simulink model "Maglev_NMPC_offsetFree"  (R2025a)
settings: Solver=ode23t  StartTime=0.0  StopTime=T_sim  FixedStep=mpc.Ts  MaxStep=0.0001  RelTol=1e-4
PreLoadFcn:
  | modelPath = fileparts(which(bdroot));
  | projectRoot = fileparts(modelPath);
  | 
  | run(fullfile(projectRoot, 'setup_sim_params.m'));
  | load(fullfile(projectRoot, 'Controller_Params', 'LKFData.mat'));
  | load(fullfile(projectRoot, 'Controller_Params', 'OffsetFreeNMPCData.mat'));
  | % Add the generated code folder so Simulink can find the mexw64
  | addpath(fullfile(projectRoot, 'Controller_Design/design_nmpc_offsetfree/c_generated_code'))
  | addpath(fullfile(projectRoot, 'Controller_Design/design_nmpc_offsetfree/c_generated_code/MaglevAug_model'))
  | 
  | load('sfun_port_names')
undefined symbols (not defined in the file): airgap_soll, Ext_Fina_Val, Ext_Init_Val, grav, I_max, I_min, lkf_params, mass, nmpc, T_stp
libraries: fl_lib x11, nesl_utility x4
settings Model: Creator=Polarstern  LastModifiedBy=CelestialAurora

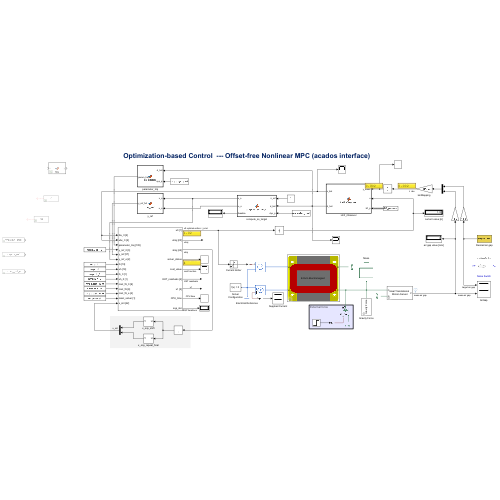
[thumbnail: Simulink's stored preview of the top-level diagram]
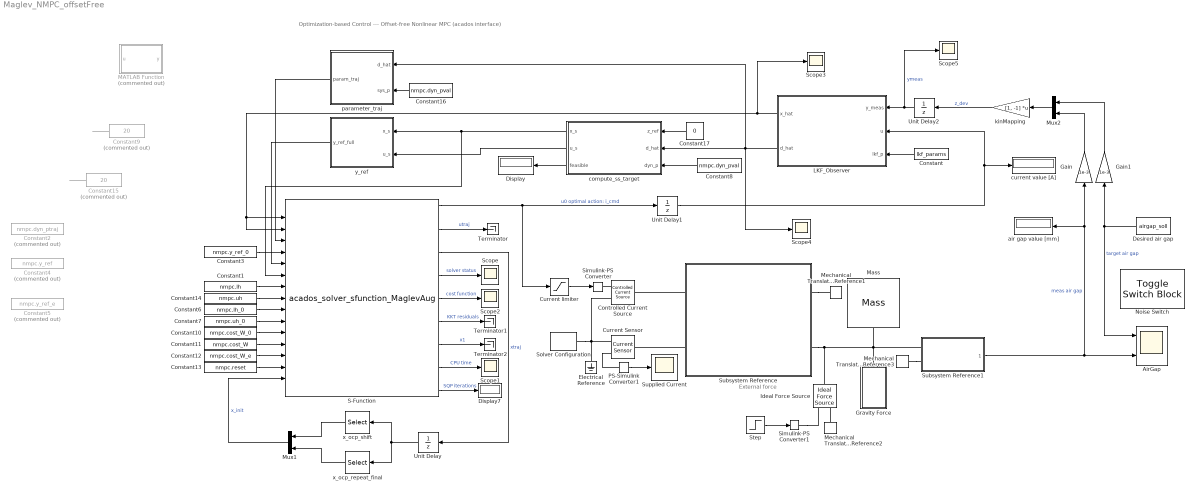
== system Maglev_NMPC_offsetFree ==
  note: Optimization-based Control --- Offset-free Nonlinear MPC (acados interface)
  note: External force
  AirGap : Scope  NumInputPorts=2
      settings: ActiveDisplayYMinimum=-0.31249999999999994  ActiveDisplayYMaximum=2.8125
  Constant : Constant  Value=lkf_params  OutDataTypeStr=Bus: lkf_Bus
  Constant1 : Constant  Value=nmpc.lh
  Constant10 : Constant  Value=nmpc.cost_W_0
  Constant11 : Constant  Value=nmpc.cost_W
  Constant12 : Constant  Value=nmpc.cost_W_e
  Constant13 : Constant  Value=nmpc.reset
  Constant14 : Constant  Value=nmpc.uh
  Constant15 : Constant  Commented=on  Value=20
  Constant16 : Constant  Value=nmpc.dyn_pval
  Constant17 : Constant  Value=0
  Constant2 : Constant  Commented=on  Value=nmpc.dyn_ptraj
  Constant3 : Constant  Value=nmpc.y_ref_0
  Constant4 : Constant  Commented=on  Value=nmpc.y_ref
  Constant5 : Constant  Commented=on  Value=nmpc.y_ref_e
  Constant6 : Constant  Value=nmpc.lh_0
  Constant7 : Constant  Value=nmpc.uh_0
  Constant8 : Constant  Value=nmpc.dyn_pval
  Constant9 : Constant  Commented=on  Value=20
  Controlled Current Source : fl_lib/Electrical/Electrical Sources/Controlled Current Source
  Current Sensor : fl_lib/Electrical/Electrical Sensors/Current Sensor
  Current limiter : Saturate  UpperLimit=I_max  LowerLimit=I_min
  Desired air gap : Constant  Value=airgap_soll
  Display : Display
  Display7 : Display
  Electrical Reference : fl_lib/Electrical/Electrical Elements/Electrical Reference
  Gain : Gain  Gain=1e-3
  Gain1 : Gain  Gain=1e-3
  Gravity Force : Subsystem
      mask DialogControl DescGroupVar Prompt: Gravity Force
      mask DialogControl DescTextVar Prompt: Fg = Mass*grav, as constant parameters predefined
      mask DialogControl DescTextVar2 Prompt: Direction: Downward
      mask Display: disp("Gravity Force")
  Ideal Force Source : fl_lib/Mechanical/Mechanical Sources/Ideal Force Source
  LKF_Observer : MATLAB Function  TreatAsAtomicUnit=on
  MATLAB Function : MATLAB Function  Commented=on  TreatAsAtomicUnit=on
  Mass : fl_lib/Mechanical/Translational Elements/Mass  mass=mass kg  num_ports=foundation.enum.numPorts2.one  v_specify=on  v_priority=Low  v=0 m/s  v_nominal_specify=off  v_nominal_value=1  v_nominal_unit=m/s  f_specify=off  f_priority=None  f=0 N  f_nominal_specify=off  f_nominal_value=700  f_nominal_unit=N
  Mechanical Translational Reference1 : fl_lib/Mechanical/Translational Elements/Mechanical Translational Reference
  Mechanical Translational Reference2 : fl_lib/Mechanical/Translational Elements/Mechanical Translational Reference
  Mechanical Translational Reference3 : fl_lib/Mechanical/Translational Elements/Mechanical Translational Reference
  Mux1 : Mux  Inputs=2
  Mux2 : Mux  Inputs=2
  Noise Switch : ToggleSwitchBlock
  PS-Simulink Converter1 : nesl_utility/PS-Simulink Converter  PhysicalDomain=network_engine_domain  SubClassName=ps_output  LeftPortType=input  RightPortType=output  PseudoPeriodic=off  Frequencies=[]  VectorFormat=inherit  Unit=inherit  AffineConversion=off
  S-Function : S-Function  FunctionName=acados_solver_sfunction_MaglevAug  SFunctionDeploymentMode=off  EnableBusSupport=off
      mask Display:
      | global sfun_input_names sfun_output_names
      | for i = 1:length(sfun_input_names)
      | 	port_label('input', i, sfun_input_names{i})
      | end
      | for i = 1:length(sfun_output_names)
      | 	port_label('output', i, sfun_output_names{i})
      | end
  Scope{,1..5} (6 alike) : Scope
      Scope settings: ActiveDisplayYMinimum=-0.49999999999999989  ActiveDisplayYMaximum=4.5
      Scope1 settings: ActiveDisplayYMinimum=-0.002376549999999999  ActiveDisplayYMaximum=0.029782950000000002  DataLoggingVariableName=ScopeData2
      Scope2 settings: ActiveDisplayYMinimum=-1  ActiveDisplayYMaximum=1  DataLoggingVariableName=ScopeData4
      Scope3 settings: ActiveDisplayYMinimum=-0.12370605676276082  ActiveDisplayYMaximum=0.39152289519586231  DataLoggingVariableName=ScopeData5
      Scope4 settings: ActiveDisplayYMinimum=-1.3296662204714107  ActiveDisplayYMaximum=0.14858706613408232  DataLoggingVariableName=ScopeData6
      Scope5 settings: ActiveDisplayYMinimum=-0.00081250000000000007  ActiveDisplayYMaximum=0.0023125000000000003  DataLoggingVariableName=ScopeData7
  Simulink-PS Converter : nesl_utility/Simulink-PS Converter  PhysicalDomain=network_engine_domain  SubClassName=ps_input  LeftPortType=input  RightPortType=output  PseudoPeriodic=off  Frequencies=[]  NoiseDistribution=none  NoiseParameters=[]  Unit=1  AffineConversion=off  FilteringAndDerivatives=zero  SimscapeFilterOrder=1  InputFilterTimeConstant=0.001  UdotUserProvided=0
  Simulink-PS Converter1 : nesl_utility/Simulink-PS Converter  PhysicalDomain=network_engine_domain  SubClassName=ps_input  LeftPortType=input  RightPortType=output  PseudoPeriodic=off  Frequencies=[]  NoiseDistribution=none  NoiseParameters=[]  Unit=1  AffineConversion=off  FilteringAndDerivatives=provide  SimscapeFilterOrder=1  InputFilterTimeConstant=0.001  UdotUserProvided=0
  Solver Configuration : nesl_utility/Solver Configuration  PhysicalDomain=network_engine_domain  SubClassName=solver  LeftPortType=input  RightPortType=generic  Tones=[]  Harmonics=[]  SimulateNoise=off  Profile=off  UseLocalSampling=off  EnableSwitchedLinearOptims=on  FrequencyDomain=off  UseCCode=off  RelTol=0.001  AbsTol=1e-06  MinStep=1e-09  ToWorkspace=off  RevertToSquareIcSolve=off  NumHomotopyIterations=100  PhasorMode=off  PhasorModeNumHarmonics=1  ConsistencySolver=NEWTON_XTOL_AFTER_FTOL  IndexReductionMethod=DerivativeReplacement  DoDC=off  ResidualTolerance=1e-09  ConsistencyTolSource=GLOBAL  ConsistencyAbsTol=0.001  ConsistencyRelTol=0.001  ConsistencyTolFactor=0.001  UseLocalSolver=off  LocalSolverChoice=NE_BACKWARD_EULER_ADVANCER  ResolveIndetEquations=on  FunctionEvalNumThread=1  LocalSolverSampleTime=0.001  DoFixedCost=off  MaxNonlinIter=3  MaxModeIter=2  ComputeImpulses=off  ImpulseIterations=2  LinearAlgebra=auto  LinearAlgebraNumThread=0  EquationFormulation=NE_TIME_EF  DelaysMemoryBudget=1024  AutomaticFiltering=on  FilteringTimeConstant=0.001  PartitionStorageMethod=AS_NEEDED  PartitionMemoryBudget=1024  PartitionMethod=ROBUST  MultibodyUseLocalSolver=off  MultibodyLocalSolverChoice=ODE1  MultibodyLocalSolverSampleTime=0.001
  Step : Step  Time=T_stp  Before=Ext_Init_Val  After=Ext_Fina_Val  SampleTime=0
  Subsystem Reference : Subsystem  ReferencedSubsystem=IntegratedElectromagnet  l_airgap=airgap_init
  Subsystem Reference1 : Subsystem  ReferencedSubsystem=IdealTrans_MotionSensor  ns_sw=isNoiseActive  ns_pw=NoisePower  ts=Ts  init_pos=airgap_init
  Supplied Current : Scope
      settings: ActiveDisplayYMinimum=-0.5608888953934309  ActiveDisplayYMaximum=6.1901533618851614  DataLoggingVariableName=ScopeData3
  Terminator : Terminator
  Terminator1 : Terminator
  Terminator2 : Terminator
  Unit Delay : UnitDelay  InitialCondition=nmpc.x_init  SampleTime=-1  HasFrameUpgradeWarning=on
  Unit Delay1 : UnitDelay  InitialCondition=lkf_params.u_eq  SampleTime=-1  HasFrameUpgradeWarning=on
  Unit Delay2 : UnitDelay  InitialCondition=nmpc.x_init_con(1)  SampleTime=-1  HasFrameUpgradeWarning=on
  air gap value [mm] : Display
      settings: Decimation=4
  compute_ss_target : MATLAB Function  TreatAsAtomicUnit=on
  current value [A] : Display
  kinMapping : Gain  Gain=[1, -1]  Multiplication=Matrix(K*u) (u vector)
  parameter_traj : MATLAB Function  TreatAsAtomicUnit=on
  x_ocp_repeat_final : Selector  IndexMode=Zero-based  InputPortWidth=(nmpc.N+1)*nmpc.nx  IndexOptions=Starting index (dialog)  Indices=nmpc.N*nmpc.nx  OutputSizes=nmpc.nx
  x_ocp_shift : Selector  IndexMode=Zero-based  InputPortWidth=(nmpc.N+1)*nmpc.nx  IndexOptions=Starting index (dialog)  Indices=nmpc.nx  OutputSizes=nmpc.N*nmpc.nx
  y_ref : MATLAB Function  TreatAsAtomicUnit=on
  wires:
  Current limiter/1 -> Simulink-PS Converter/1
  PS-Simulink Converter1/1 -> Supplied Current/1
  S-Function/1 -> Current limiter/1, Unit Delay1/1  "u0 optimal action: i_cmd"
  S-Function/2 -> Terminator/1  "utraj"
  S-Function/3 -> Unit Delay/1  "xtraj"
  S-Function/4 -> Scope/1  "solver status"
  S-Function/5 -> Scope2/1  "cost function"
  S-Function/6 -> Terminator1/1  "KKT residuals"
  S-Function/7 -> Terminator2/1  "x1"
  S-Function/8 -> Scope1/1  "CPU time"
  S-Function/9 -> Display7/1  "SQP iterations"
  Unit Delay/1 -> x_ocp_repeat_final/1, x_ocp_shift/1
  x_ocp_repeat_final/1 -> Mux1/2
  x_ocp_shift/1 -> Mux1/1
  Step/1 -> Simulink-PS Converter1/1
  LKF_Observer/1(x_hat) -> Scope3/1, S-Function/1, S-Function/2
  Constant3/1 -> S-Function/4
  Constant1/1 -> S-Function/7
  Constant14/1 -> S-Function/8
  Constant6/1 -> S-Function/9
  Constant7/1 -> S-Function/10
  Constant10/1 -> S-Function/11
  Constant11/1 -> S-Function/12
  Constant12/1 -> S-Function/13
  Constant13/1 -> S-Function/14
  Mux1/1 -> S-Function/15  "x_init"
  Gain/1 -> Mux2/2
  Subsystem Reference1/1 -> AirGap/2, air gap value [mm]/1, Gain/1  "meas air gap"
  Desired air gap/1 -> AirGap/1, Gain1/1  "target air gap"
  kinMapping/1 -> Unit Delay2/1  "z_dev"
  Mux2/1 -> kinMapping/1
  Constant/1 -> LKF_Observer/3(lkf_p)
  LKF_Observer/2(d_hat) -> Scope4/1, parameter_traj/1(d_hat), compute_ss_target/2(d_hat)
  Constant8/1 -> compute_ss_target/3(dyn_p)
  Gain1/1 -> Mux2/1
  compute_ss_target/3(feasible) -> Display/1
  compute_ss_target/2(u_s) -> y_ref/2(u_s)
  compute_ss_target/1(x_s) -> S-Function/6, y_ref/1(x_s)
  Unit Delay2/1 -> Scope5/1, LKF_Observer/1(y_meas)  "ymeas"
  y_ref/1(y_ref_full) -> S-Function/5
  Unit Delay1/1 -> LKF_Observer/2(u), current value [A]/1
  Constant15/1 -> ?
  Constant9/1 -> ?
  Constant16/1 -> parameter_traj/2(sys_p)
  parameter_traj/1(param_traj) -> S-Function/3
  Constant17/1 -> compute_ss_target/1(z_ref)
  connections:
  Subsystem Reference/RConn2 -- Subsystem Reference1/LConn1 -- Gravity Force/RConn1 -- Mass/LConn1 -- Ideal Force Source/LConn1
  Current Sensor/RConn2 -- Controlled Current Source/RConn2 -- Solver Configuration/RConn1 -- Electrical Reference/LConn1
  Subsystem Reference/LConn1 -- Controlled Current Source/LConn1
  Subsystem Reference/LConn2 -- Current Sensor/LConn1
  Simulink-PS Converter/RConn1 -- Controlled Current Source/RConn1
  PS-Simulink Converter1/LConn1 -- Current Sensor/RConn1
  Subsystem Reference/RConn1 -- Mechanical Translational Reference1/LConn1
  Simulink-PS Converter1/RConn1 -- Ideal Force Source/RConn1
  Mechanical Translational Reference2/LConn1 -- Ideal Force Source/RConn2
  Mechanical Translational Reference3/LConn1 -- Subsystem Reference1/LConn2

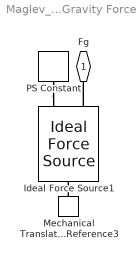
== system Maglev_NMPC_offsetFree/Gravity Force ==
  Ideal Force Source1 : fl_lib/Mechanical/Mechanical Sources/Ideal Force Source
  Mechanical Translational Reference3 : fl_lib/Mechanical/Translational Elements/Mechanical Translational Reference
  PS Constant : fl_lib/Physical Signals/Sources/PS Constant  constant=mass*grav N
  Fg : PMIOPort  Side=Right
  connections:
  Mechanical Translational Reference3/LConn1 -- Ideal Force Source1/LConn1
  PS Constant/RConn1 -- Ideal Force Source1/RConn1
  Ideal Force Source1/RConn2 -- Fg/RConn1

== matlab function Maglev_NMPC_offsetFree/compute_ss_target ==
  data: z_ref input; x_s output; d_hat input; dyn_p input; u_s output; feasible output
function [x_s, u_s, feasible] = compute_ss_target(z_ref, d_hat, dyn_p)
% COMPUTE_SS_TARGET  Analytical steady-state target for offset-free Maglev MPC
%
%  At steady-state (ẋ = 0):
%    v_s = 0                            →  xs = [z_ref; 0]
%    K/m · u_s²/(s0-z_ref)² - g + d̂ = 0  →  solve for u_s
%
%  Solving for u_s:
%    u_s = (s0 - z_ref) · √(m·(g - d̂)/K)
%
%  Physical interpretation:
%    Without mismatch (d̂=0): u_s equals the nominal equilibrium current.
%    With mismatch (d̂≠0):  u_s is adjusted so the magnetic force
%    exactly balances gravity plus the disturbance force.
%
%  If d̂ > 0  →  net upward disturbance (model under-predicts lift):
%    g_eff = g - d̂  decreases  →  u_s decreases (less current needed)
%  If d̂ < 0  →  net downward disturbance (extra load, model under-predicts gravity):
%    g_eff = g - d̂  increases  →  u_s increases (more current needed)
%
%  Inputs:
%    z_ref   reference position      [m]
%    d_hat   estimated disturbance   [m/s²]  (from LKF observer)
%    dyn_p   dynamic parameters: [K, m, s0, g]
%         - K     % magnetic constant       [N·m²/A²]  
%         - m     % mass                    [kg]
%         - s0    % air gap reference       [m]
%         - g     % gravity                 [m/s²]
%
%  Outputs:
%    x_s      [2×1]  steady-state state  [z_ref; 0]
%    u_s      [1×1]  steady-state current [A]  (clamped to [0, 15] A)
%    feasible [bool] false if physical limits violated

K  = dyn_p(1);    
m  = dyn_p(2);    
s0 = dyn_p(3);    
g  = dyn_p(4);    

x_s = [z_ref; 0];
feasible = true;

% --- Guard 1: position must be inside the air gap ---
gap_ref = s0 - z_ref;
if gap_ref <= 0 || gap_ref >= s0    % physical gap must be in (0, s0)
    u_s = 0; feasible = false; return
end

% --- Guard 2: effective gravity must remain positive ---
g_eff = g - d_hat;
if g_eff <= 0
    warning('compute_ss_target: g_eff = g - d_hat = %.4f <= 0. Clamping.', g_eff);

    g_eff = 1e-3;   % safety floor
    feasible = false;
end

% --- Analytical solution ---
u_s = (s0 - z_ref) * sqrt(m * g_eff / K);

% --- Clamp to actuator limits ---
I_min = 0;  I_max = 15;
if u_s < I_min || u_s > I_max
    feasible = false;
end
u_s = max(I_min, min(I_max, u_s));

end

== matlab function Maglev_NMPC_offsetFree/LKF_Observer ==
  data: y_meas input; u input; x_hat output; d_hat output; lkf_p input
function [x_hat, d_hat] = LKF_Observer(y_meas, u, lkf_p) 
% LKF_OBSERVER  Single-function predict-correct Kalman step for the
%               augmented state [z; v; d].
%
%  LKF cycle at step k:
%    Stored state : x_aug_pred = x̂_{k|k-1}  (from previous step)
%
%    CORRECTION  (measurement update):
%      innovation = y_k  -  Cd · x̂_{k|k-1}
%      x̂_{k|k}   = x̂_{k|k-1}  +  L_kf · innovation
%
%    PREDICTION  (time update):
%      x̂_{k+1|k} = Ad · x̂_{k|k}  +  Bd · u_k
%
%  INPUTS
%    y_meas  [1×1]   measured position at step k      [m]
%    u       [1×1]   control input applied at step k  [A]
%    lkf_p   struct  fields: Ad [3×3], Bd [3×1], Cd [1×3], L_kf [3×1]
%
%  OUTPUTS
%    x_hat   [2×1]   corrected state estimate [z_hat; v_hat]
%    d_hat   [1×1]   corrected disturbance estimate d̂_k

persistent x_aug_pred   % x̂_{k|k-1} stored between steps
v_sat = 0.34; s0 = 0.002;
%% Initialise on first call
if isempty(x_aug_pred)
    x_aug_pred = [y_meas; 0; 0];   % z from sensor, v = 0, d = 0
end

% Explicitly enforce dimensions — Bus signals can silently collapse 2D arrays
Ad_ = reshape(lkf_p.Ad,   3, 3);      % [3×3]
Bd_ = reshape(lkf_p.Bd,   3, 1);      % [3×1]
Cd_ = reshape(lkf_p.Cd,   1, 3);      % [1×3]
Lk_ = reshape(lkf_p.L_kf, 3, 1);      % [3×1]

%% CORRECTION  (measurement update)
innovation   = y_meas - Cd_ * x_aug_pred;
x_aug_corr   = x_aug_pred + Lk_ * innovation;          % x̂_{k|k}

% Clip disturbance to physically plausible range (anti-windup)
x_aug_corr(3) = max(-0.9*9.81, min(0.9*9.81, x_aug_corr(3)));
x_aug_corr(2) = max(-v_sat, min(v_sat, x_aug_corr(2)));

d_hat = x_aug_corr(3);   % feed corrected d̂ to SS target calculator

%% PREDICTION  (time update)
delta_u    = u - lkf_p.u_eq; 
x_aug_pred = Ad_ * x_aug_corr + Bd_ * delta_u;              % x̂_{k+1|k} → stored

% Clamp predicted position to physical range   ← ADD THIS
x_aug_pred(1) = max(-s0, min(s0, x_aug_pred(1)));

%% Outputs
x_hat = x_aug_corr(1:2);   % [z_hat; v_hat]

end

== matlab function Maglev_NMPC_offsetFree/y_ref ==
  data: x_s input; y_ref_full output; u_s input
function y_ref_full = tile_yref(x_s, u_s)

    % N  = coder.const(mpc_p.N);    % compile-time constant from struct port
    N = 20;
    y_ref_full = repmat([x_s; u_s], N-1, 1);   % (N·ny) × 1
    
end

== matlab function Maglev_NMPC_offsetFree/MATLAB Function ==
  data: u input; y output
function y = fcn(u)
    % In Simulink: use a Memory + Switch block, or inside the function:
    persistent u_s_last
    if isempty(u_s_last), u_s_last = u_eq; end
    if ~feasible
        u_s = u_s_last;   % hold last good value
    else
        u_s_last = u_s;
    end
y = u;

== matlab function Maglev_NMPC_offsetFree/parameter_traj ==
  data: d_hat input; param_traj output; sys_p input
function param_traj = tile_params(d_hat, sys_p)

    N  = 20; %coder.const(N);    % horizon
    % np = coder.const(sys_p);   % number of parameters = 5
    
    p_stage  = [sys_p; d_hat];  % 5×1
    param_traj = repmat(p_stage, N+1, 1);   % (N+1)·np × 1
end
